simulink model "BOOst_mppt"  (R2022a)
settings: Solver=VariableStepAuto  StartTime=0.0  StopTime=0.1  RelTol=1e-3
InitFcn:
  | Vg=250;
  | Vo=800;
  | L=1.1e-3;
  | C=900e-6;
  | D=(1-250/800);
  | R=150;
  | IL=6;
  | 
  | %statefunction
  | AS=[0 -(1-D)/L;(1-D)/C -1/(R*C)];
  | BS=[1/L 0 Vo/L;0 -1/C -IL/C];
  | CS=[0 1;1 0];
  | DS=[0 0 0;0 0 0];
libraries: spsSeriesRLCBranchLib x3, spsControlledVoltageSourceLib x1, spsDiodeLib x1, spsIGBTLib x1, spsPWMGeneratorDCDCLib x1, spsVoltageMeasurementLib x1, spspowerguiLib x1
settings Model: Creator=jeffr  LastModifiedBy=jeffr
settings SolverCC: ZeroCrossAlgorithm=Adaptive
settings DebuggingCC: IgnoredZcDiagnostic=none

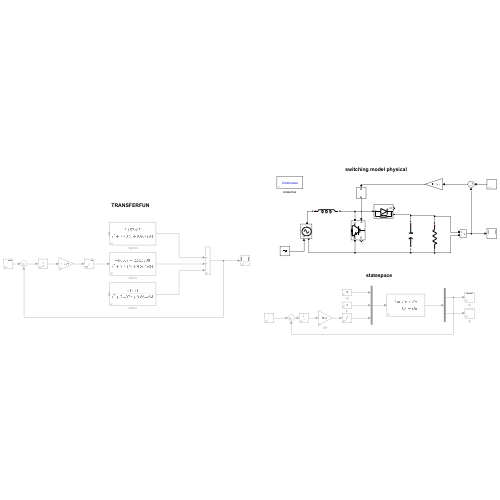
[thumbnail: Simulink's stored preview of the top-level diagram]
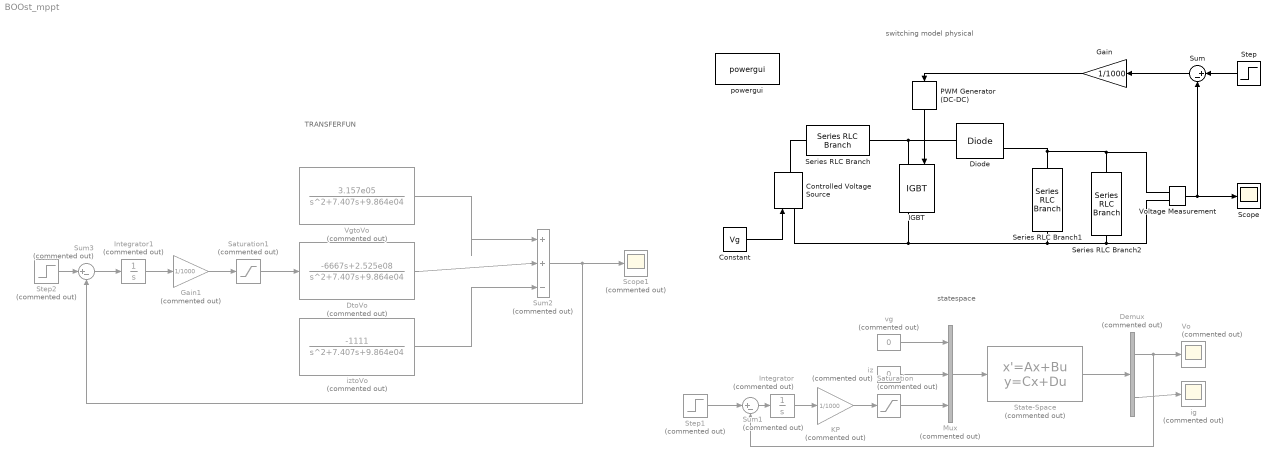
== system BOOst_mppt ==
  note: switching model physical
  note: statespace
  note: TRANSFERFUN
  Constant : Constant  Value=Vg
  Controlled Voltage Source : spsControlledVoltageSourceLib/Controlled Voltage Source  Initialize=on  Source_Type=DC  Amplitude=0  Phase=0  Frequency=0  Measurements=None
  Demux : Demux  Commented=on  Outputs=2
  Diode : spsDiodeLib/Diode  Ron=0.001  Lon=0  Vf=0.8  IC=0  UseSnubber=0  Rs=500  Cs=250e-9  Measurements=on
  DtoVo : TransferFcn  Commented=on  Numerator="[-6667  2.525e08]"  Denominator="[1 7.407  9.864e04]"
  Gain : Gain  Gain=1/1000
  Gain1 : Gain  Commented=on  Gain=1/1000
  IGBT : spsIGBTLib/IGBT  Ron=0.001  Lon=0  Vf=1  Tf=1e-6  Tt=2e-6  IC=0  Rs=1e5  Cs=inf  Measurements=on
  Integrator : Integrator  Commented=on
  Integrator1 : Integrator  Commented=on
  KP : Gain  Commented=on  Gain=1/1000
  Mux : Mux  Commented=on  Inputs=3
  PWM Generator (DC-DC) : spsPWMGeneratorDCDCLib/PWM Generator (DC-DC)  Fsw=100000  Ts=0
  Saturation : Saturate  Commented=on
  Saturation1 : Saturate  Commented=on  UpperLimit=1  LowerLimit=0
  Scope : Scope
  Scope1 : Scope  Commented=on
  Series RLC Branch : spsSeriesRLCBranchLib/Series RLC Branch  LConnTagsString=__new0  RConnTagsString=__new0  BranchType=L  Resistance=1  Inductance=L  SetiL0=off  InitialCurrent=0  Capacitance=1e-6  Setx0=off  InitialVoltage=0  Measurements=None
  Series RLC Branch1 : spsSeriesRLCBranchLib/Series RLC Branch  LConnTagsString=__new0  RConnTagsString=__new0  BranchType=C  Resistance=1  Inductance=L  SetiL0=off  InitialCurrent=0  Capacitance=C  Setx0=off  InitialVoltage=0  Measurements=None
  Series RLC Branch2 : spsSeriesRLCBranchLib/Series RLC Branch  LConnTagsString=__new0  RConnTagsString=__new0  BranchType=R  Resistance=R  Inductance=L  SetiL0=off  InitialCurrent=0  Capacitance=C  Setx0=off  InitialVoltage=0  Measurements=None
  State-Space : StateSpace  Commented=on  A=AS  B=BS  C=CS  D=DS  InitialCondition=0
  Step : Step  Time=10  Before=800  After=800  SampleTime=0
  Step1 : Step  Commented=on  Time=5  Before=1  After=800  SampleTime=0
  Step2 : Step  Commented=on  Time=5  Before=800  After=800  SampleTime=0
  Sum : Sum  Inputs=|+-
  Sum1 : Sum  Commented=on  Inputs=|+-
  Sum2 : Sum  Commented=on  Inputs=|++-
  Sum3 : Sum  Commented=on  Inputs=|+-
  VgtoVo : TransferFcn  Commented=on  Numerator=[3.157e05]  Denominator="[1 7.407  9.864e04]"
  Vo : Scope  Commented=on
  Voltage Measurement : spsVoltageMeasurementLib/Voltage Measurement  PhasorSimulation=off  OutputType=Complex  PSBequivalent=0
  ig : Scope  Commented=on
  iz : Constant  Commented=on  Value=0
  iztoVo : TransferFcn  Commented=on  Numerator=[-1111]  Denominator="[1 7.407  9.864e04]"
  powergui : spspowerguiLib/powergui  Priority=1  SimulationMode=Continuous  SampleTime=50e-6  frequency=60  Iterations=50  frequencyindice=0  Pbase=100e6  ErrMax=1e-4  UnitsV=kV  UnitsW=MW  buscounter=0  FunctionMessages=off  echomessages=off  EnableUseOfTLC=off  CurrentSourceSwitches=off  DisableSnubberDevices=off  DisableRonSwitches=off  DisableVfSwitches=off  DisplayEquations=off  AutomaticDiscreteSolvers=off  SolverType=Tustin/Backward Euler (TBE)  Interpol=off  ExternalGateDelay=off  methode=off  Ts=100  x0status=blocks  SPID=on  SwTol=0  HookPort=off  NonlinearTolerance=1e-4  nMaxIteration=100  ContinueOnMaxIteration=off  RestoreLinks=warning  ResistiveCurrentMeasurement=off  Frange=[0:2:500]  Ylog=off  Xlog=on  ShowGrid=off  save=off  variable=ZData  structure=0  ZoomFFT=off  StartTime=0.0  cycles=1  DisplayStyle=1  fundamental=60  FreqAxis=off  MaxFrequency=1000  frequencyindicesteady=1  RmsSteady=1  display=off
  vg : Constant  Commented=on  Value=0
  wires:
  Voltage Measurement/1 -> Scope/1, Sum/2
  Constant/1 -> Controlled Voltage Source/1
  PWM Generator (DC-DC)/1 -> IGBT/1
  Step/1 -> Sum/1
  Sum/1 -> Gain/1
  Mux/1 -> State-Space/1
  vg/1 -> Mux/1
  iz/1 -> Mux/2
  Saturation/1 -> Mux/3
  KP/1 -> Saturation/1
  State-Space/1 -> Demux/1
  Demux/1 -> Vo/1, Sum1/2
  Demux/2 -> ig/1
  Step1/1 -> Sum1/1
  Sum1/1 -> Integrator/1
  Integrator/1 -> KP/1
  VgtoVo/1 -> Sum2/1
  DtoVo/1 -> Sum2/2
  iztoVo/1 -> Sum2/3
  Sum3/1 -> Integrator1/1
  Step2/1 -> Sum3/1
  Integrator1/1 -> Gain1/1
  Gain1/1 -> Saturation1/1
  Saturation1/1 -> DtoVo/1
  Sum2/1 -> Scope1/1, Sum3/2
  Gain/1 -> PWM Generator (DC-DC)/1
  connections:
  Controlled Voltage Source/RConn1 -- Series RLC Branch/LConn1
  Series RLC Branch/RConn1 -- Diode/LConn1 -- IGBT/LConn1
  Series RLC Branch1/LConn1 -- Voltage Measurement/LConn1 -- Series RLC Branch2/LConn1 -- Diode/RConn1
  Controlled Voltage Source/LConn1 -- IGBT/RConn1 -- Voltage Measurement/LConn2 -- Series RLC Branch2/RConn1 -- Series RLC Branch1/RConn1
